simulink model "Bungee"  (R2023b)
settings: Solver=VariableStepAuto  StartTime=0.0  StopTime=100  RelTol=1e-3
settings Model: Creator=Andrei  LastModifiedBy=mateisorodoc

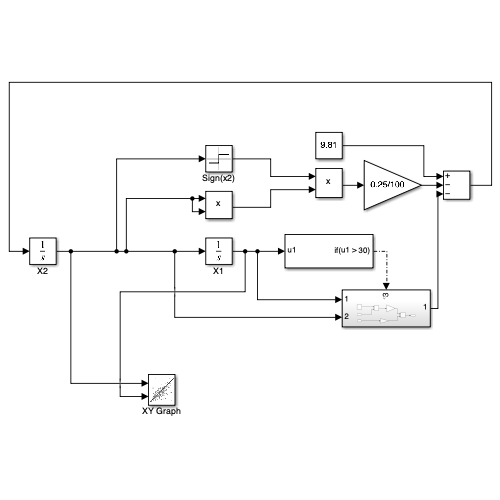
[thumbnail: Simulink's stored preview of the top-level diagram]
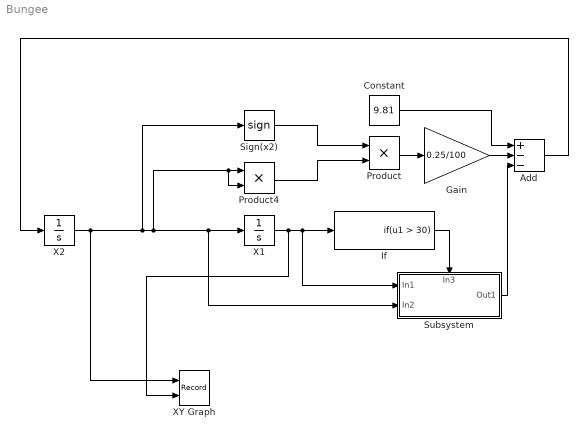
== system Bungee ==
  Add : Sum  Inputs=+--
  Constant : Constant  Value=9.81
  Gain : Gain  Gain=0.25/100
  If : If  IfExpression=u1 > 30  ShowElse=off
  Product : Product
  Product4 : Product
  Sign(x2) : Signum
  Subsystem : Subsystem
      settings: PortSchema="{\"entries\":[{\"content\":{\"sides\":[{\"content\":{\"connectorIds\":[\"In1\",\"In2\"]},\"type\":\"ConnectorPlacement.EquallySpacedRectSide\",\"uuid\":\"98daaf6b-24fb-418d-8748-a759574185a5\"},{\"content\":{\"connectorIds\":[\"Out1\"],\"side\":\"RIGHT\"},\"type\":\"ConnectorPlacement.EquallySpacedRectSide\",\"uuid\":\"e91c8372-d3c1-4254-b2f2-5c5618fd172c\"},{\"content\":{\"connectorIds\":[\"In3\"],\"side\":\"TOP\"},\"type\":\"ConnectorPlacement.EquallySpacedRectSide\",\"uuid\":\"8b08129d-9da4-43b6-b5fb-a4f05161936c\"},{\"content\":{\"side\":\"BOTTOM\"},\"type\":\"ConnectorPlacement.EquallySpacedRectSide\",\"uuid\":\"9b0ce049-0b03-44fd-9b11-d851291cbb6f\"}]},\"type\":\"ConnectorPlacement.EquallySpacedConnector\",\"uuid\":\"57f4f152-05cf-4879-a0f8-46c61caa10d0\"}],\"packageUris\":[\"http://schema.mathworks.com/mf0/Connector/R2020b\"],\"version\":\"1.0\"}"
  X1 : Integrator
  X2 : Integrator
  XY Graph : Record  FileSettingsInternal="{\"entries\":[{\"content\":{\"excelSettings\":{\"content\":{},\"type\":\"Streamout.ExcelSettings\"}},\"type\":\"Streamout.FileSettingStorage\",\"uuid\":\"\"}],\"packageUris\":[\"http:\\/\\/schema.mathworks.com\\/mf0\\/streamout_blocks\\/R2020a\"],\"version\":\"1.0\"}"  Layout=[1 1]  SignalsInternal="{\"entries\":[{\"content\":{\"signals\":[{\"content\":{\"blockPath\":[],\"dimensions\":[1],\"domain\":\"\",\"lineColor\":\"#a2142f\",\"plots\":[1],\"port\":1,\"sid\":[\"\"],\"signalID\":198,\"signalName\":\"X2\"},\"type\":\"RecordBlkView.Signal\",\"uuid\":\"\"},{\"content\":{\"blockPath\":[],\"dimensions\":[1],\"domain\":\"\",\"lineColor\":\"#139fff\",\"plots\":[1],\"port\":2,\"sid\":[\"\"],\"signalID\":202,\"signalName\":\"X1\"},\"type\":\"RecordBlkView.Signal\",\"uuid\":\"\"}]},\"type\":\"RecordBlkView.InputSignals\",\"uuid\":\"\"}],\"packageUris\":[\"http:\\/\\/schema.mathworks.com\\/mf0\\/streamout_blocks\\/R2020a\"],\"version\":\"1.0\"}"  VisualizationBindings="{\"xyplotplugin\":{\"info\":[{\"series\":[{\"bindingParametersList\":[{\"parameter\":\"X-Axis\",\"signalID\":198,\"signalName\":\"X2\"},{\"parameter\":\"Y-Axis\",\"signalID\":202,\"signalName\":\"X1\"}],\"seriesID\":24141}],\"subplotID\":1}]}}"  CompatibilityTag=XY  st=-1
  wires:
  X2/1 -> XY Graph/1, Sign(x2)/1, Product4/2, Product4/1, Subsystem/2(In2), X1/1
  Product4/1 -> Product/2
  Constant/1 -> Add/1
  Sign(x2)/1 -> Product/1
  Gain/1 -> Add/2
  Product/1 -> Gain/1
  X1/1 -> XY Graph/2, Subsystem/1(In1), If/1
  If/1 -> Subsystem/3(In3)
  Subsystem/1(Out1) -> Add/3
  Add/1 -> X2/1

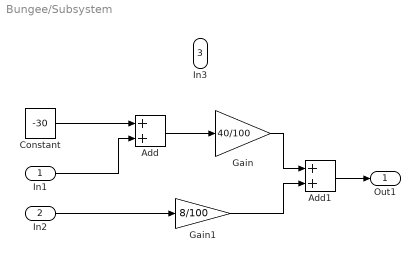
== system Bungee/Subsystem ==
  In1 : Inport
  In2 : Inport  Port=2
  In3 : Inport  Port=3
  Add : Sum
  Add1 : Sum
  Constant : Constant  Value=-30
  Gain : Gain  Gain=40/100
  Gain1 : Gain  Gain=8/100
  Out1 : Outport
  wires:
  In1/1 -> Add/2
  Constant/1 -> Add/1
  Add/1 -> Gain/1
  In2/1 -> Gain1/1
  Gain/1 -> Add1/1
  Gain1/1 -> Add1/2
  Add1/1 -> Out1/1
